simulink model "follow_right_hand"  (Simulink 8.7)
settings: Solver=FixedStepAuto  StartTime=0.0  StopTime=inf  FixedStep=0.01  RelTol=1e-3
settings Model: Creator=maximilian  LastModifiedBy=eispin
settings DataIOCC: LimitDataPoints=off  SaveFormat=Dataset
settings DebuggingCC: UnderspecifiedInitializationDetection=Simplified  MergeDetectMultiDrivingBlocksExec=error
settings HardwareCC: ProdBitPerPointer=64  ProdLargestAtomicFloat=Float  ProdIntDivRoundTo=Zero  ProdEndianess=LittleEndian  ProdWordSize=64  ProdHWDeviceType=Intel->x86-64 (Windows64)
settings ModelReferenceCC: PropagateSignalLabelsOutOfModel=on
settings ConfigComp: CovModelRefEnable=off

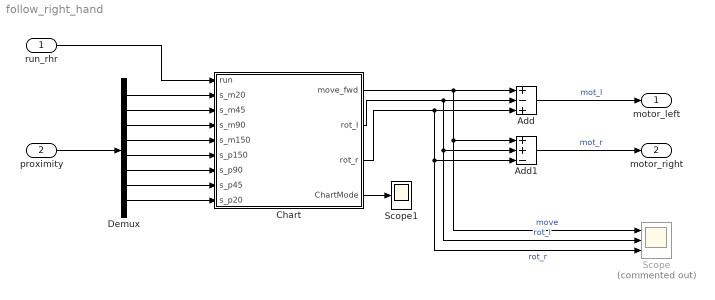
== system follow_right_hand ==
  run_rhr : Inport
  proximity : Inport  Port=2  PortDimensions=[8]
  Add : Sum  Inputs=+-+
  Add1 : Sum  Inputs=++-
  Chart : Stateflow chart  TreatAsAtomicUnit=on
  Demux : Demux  Outputs=8
  Scope : Scope  Commented=on  NumInputPorts=3
  Scope1 : Scope
  motor_left : Outport
  motor_right : Outport  Port=2
  wires:
  Demux/1 -> Chart/2(s_m20)
  Demux/2 -> Chart/3(s_m45)
  Demux/3 -> Chart/4(s_m90)
  Demux/4 -> Chart/5(s_m150)
  Demux/5 -> Chart/6(s_p150)
  Demux/6 -> Chart/7(s_p90)
  Demux/7 -> Chart/8(s_p45)
  Demux/8 -> Chart/9(s_p20)
  proximity/1 -> Demux/1
  Chart/2(rot_l) -> Scope/2, Add1/2, Add/2  "rot_l"
  Chart/3(rot_r) -> Scope/3, Add1/3, Add/3  "rot_r"
  Chart/1(move_fwd) -> Scope/1, Add1/1, Add/1  "move"
  Add1/1 -> motor_right/1  "mot_r"
  Add/1 -> motor_left/1  "mot_l"
  Chart/4(ChartMode) -> Scope1/1
  run_rhr/1 -> Chart/1(run)

== stateflow chart Chart ==
  state findWall
    entry:
    move_fwd=mv_per_sec;
    rot_l = 0;
    rot_r = 0;
  state checkWall
    % known: nothing
    entry:
    move_fwd = 0;
    rot_r = 0;
    rot_l = 0;
    [wall_p wall_rot] = find_wall([s_m150, s_m90, s_m45, s_m20, s_p20, s_p45, s_p90, s_p150]);
  state wallWaiter
  state claustrophobia
    % known: have -20, -45, -90
    entry:
    move_fwd = 0;
    rot_l = 0;
    rot_r = 0;
  state avoidCollision
    % known: have -20, -45
    entry:
    move_fwd = 0;
    rot_l = 0;
    rot_r = 0;
  state orientToWall
    % known: have -20
    entry:
    move_fwd = mv_per_sec;
    rot_r = 0;
    rot_l = 0;
  state follow
    % known: have -45, -90
    entry:
    move_fwd = mv_per_sec;
    rot_l = 0;
    rot_r = 0;
  state runClose
    % known: (should) have -45
    entry:
    move_fwd = mv_per_sec;
    rot_l = 0;
    rot_r = 0;
  note: => Move roughly sin(44 degree)*(x length unit) towards straight wall
      | => if we just drifted away, that's all we need to find the wall again
  state stayClose
    % known: have -90, NOT have -45
    entry:
    move_fwd = 0;
    rot_l = 0;
    rot_r = 0;
  state goOn
  note: => Move roughly sin(5 degree)*(4 length units) away from straight wall
  (default) -> checkWall
  checkWall -> findWall [order 4] : [wall_p == 0]
  findWall -> checkWall : [s_m45 <= sens_tol || s_m20 <= sens_tol || s_p45 <= sens_tol || s_p20 <= sens_tol]
  checkWall -> orientToWall [order 3] : [wall_p == 1 && wall_rot == 0]
  checkWall -> wallWaiter [order 2] : [wall_p == 1 && wall_rot > 0]{rot_l = 1;}
  checkWall -> wallWaiter [order 1] : [wall_p == 1 && wall_rot <= 0]{rot_r = 1; wall_rot = -wall_rot;}
  wallWaiter -> orientToWall : [after(wall_rot*(pi/180)/rot_per_sec, sec)]
  claustrophobia -> follow : [s_m20 > sens_tol && after(5*(pi/180)/rot_per_sec,sec)]
  orientToWall -> avoidCollision : [s_m45 <= sens_tol]
  avoidCollision -> claustrophobia [order 2] : [s_m90 <= sens_tol]
  avoidCollision -> orientToWall [order 1] : [s_m45 > sens_tol && after(5*(pi/180)/rot_per_sec, sec)]
  goOn -> claustrophobia [order 2] : [s_m20 <= sens_tol]
  follow -> claustrophobia [order 1] : [s_m20 <= sens_tol]
  runClose -> orientToWall [order 1] : [s_m20 <= sens_tol]
  goOn -> follow [order 3] : [s_m45 <= sens_tol]
  runClose -> stayClose [order 2] : [s_m45 > sens_tol && after(0.6/mv_per_sec, sec)]
  follow -> goOn [order 2] : [s_m45 > sens_tol]
  stayClose -> runClose : [after(44*(pi/180)/rot_per_sec, sec)]
  goOn -> stayClose [order 1] : [after(4/mv_per_sec, sec)]
  data: run input double; s_m20 input double; s_m45 input double; move_fwd output double; rot_l output double; rot_r output double; s_m90 input double; s_m150 input double; s_p150 input double; s_p90 input double; s_p45 input double; s_p20 input double; sens_tol constant double =7; rot_per_sec constant double =2/5.3; mv_per_sec constant double =2; ChartMode output Enum: ChartModeType1; wall_rot local double; wall_p local double
